simulink model "GFo_29bus"  (R2015b)
settings: Solver=ode1  StartTime=0.0  StopTime=4.5  FixedStep=Time_Step  RelTol=1e-3
PreLoadFcn:
  | Init_29bus;
InitFcn:
  | Init_29bus;
undefined symbols (not defined in the file): C_line, D1, D11, Delta, DX_DR, fb, fn, I_thresh_pu, Kp_Rvi_pu, Time_Step, VSC01_Cf, VSC01_Cf_pu, VSC01_Delta_P_Time_Step, VSC01_Delta_P_Value, VSC01_id0, VSC01_Lf, VSC01_Lf_pu, VSC01_Lt_pu, VSC01_mp1, VSC01_mp2, VSC01_mp3, VSC01_Pn, VSC01_R, VSC01_Rf, VSC01_Rf_pu, VSC01_Rt_pu, VSC01_Rv, VSC01_Sn, VSC01_T1, VSC01_T2, VSC01_Tr_PLL, VSC01_Udc_n, VSC01_Udcb, VSC01_Un1, VSC01_Un2, VSC01_W_LF, VSC01_wc1, VSC01_wc2, VSC01_wc3
libraries: powerlib x183, sps_avr x6, simulink x4, powerlib_meascontrol x2
(part 5 of 6)

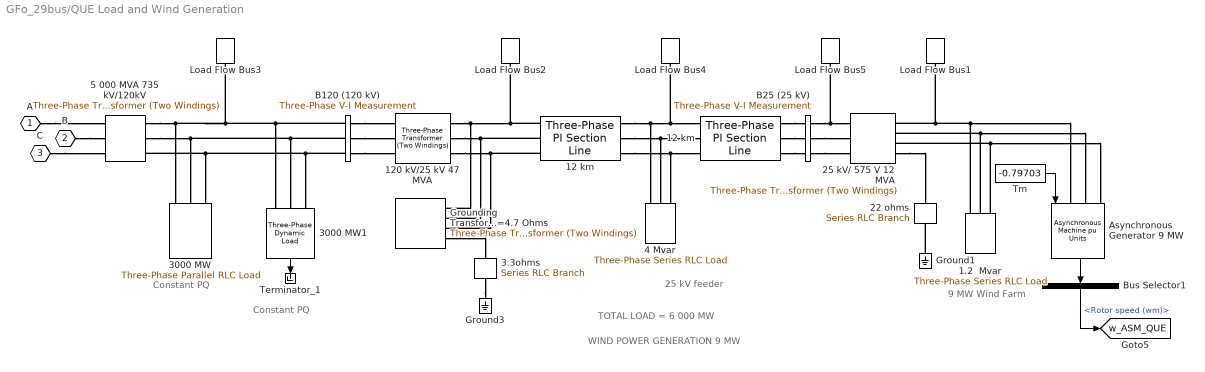
== system GFo_29bus/QUE Load and Wind Generation ==
  note: 9 MW Wind Farm
  note: 25 kV feeder
  note: Constant PQ
  note: Constant PQ
  note: WIND POWER GENERATION 9 MW
  note: TOTAL LOAD = 6 000 MW
  1.2  Mvar : powerlib/Elements/Three-Phase Series RLC Load  LConnTagsString=A|B|C  Configuration=Delta  NominalVoltage=575  Vabc=[1e3 1e3 1e3]  Vabcp=[1e3 1e3 1e3]  NominalFrequency=60  UnbalancedPower=off  ActivePower=1.2e6/50  InductivePower=0  CapacitivePower=1.2e6  Pabc=[10e3 9e3 11e3]  QLabc=[100 90 110]  QCabc=[100 90 110]  Pabcp=[10e3 9e3 11e3]  QLabcp=[100 90 110]  QCabcp=[100 90 110]  Measurements=None  LoadType=constant Z
  12 km : powerlib/Elements/Three-Phase PI Section Line  LConnTagsString=a|b|c  RConnTagsString=A|B|C  Frequency=60  Resistances=[0.1153 0.413]  Inductances=[1.05e-3 3.32e-3]  Capacitances=[11.33e-009 5.01e-009]  Length=12
  "12 km " : powerlib/Elements/Three-Phase PI Section Line  LConnTagsString=a|b|c  RConnTagsString=A|B|C  Frequency=60  Resistances=[0.1153 0.413]  Inductances=[1.05e-3 3.32e-3]  Capacitances=[11.33e-009 5.01e-009]  Length=12
  120 kV/25 kV 47 MVA : powerlib/Elements/Three-Phase Transformer (Two Windings)  Winding1Connection=Yg  Winding2Connection=Delta (D1)  CoreType=Three single-phase transformers  SetSaturation=off  Hysteresis=off  DataFile='basic_model'  SetInitialFlux=off  Measurements=None  UNITS=pu  NominalPower=[47e6 60 ]  Winding1="[ 120e3  0.08/30   0.08 ]"  Winding2="[ 25e3  0.08/30  0.08]"  Rm=500  Lm=500  L0=0.5  Saturation="[ 0,0  ;  0.005,1.2  ;  1.0,1.4 ]"  InitialFluxes=[ 0.8 , -0.8 , 0.7 ]  MoreParameters=off  BreakLoop=off  DataType=off  TransfoNumber=0
  "22 ohms " : powerlib/Elements/Series RLC Branch  LConnTagsString=__new0  RConnTagsString=__new0  BranchType=R  Resistance=22  Inductance=1.0  SetiL0=off  InitialCurrent=0  Capacitance=1.0  Setx0=off  InitialVoltage=0  Measurements=None
  25 kV/ 575 V 12 MVA : powerlib/Elements/Three-Phase Transformer (Two Windings)  Winding1Connection=Yg  Winding2Connection=Yn  CoreType=Three single-phase transformers  SetSaturation=off  Hysteresis=off  DataFile='hysteresis'  SetInitialFlux=off  Measurements=None  UNITS=pu  NominalPower="[12e6  60]"  Winding1=[25e3 , 0.025/30 , 0.025]  Winding2=[ 575, 0.025/30 , 0.025]  Rm=500  Lm=inf  L0=0.5  Saturation=[ 0,0 ; 0.0024,1.2 ; 1.0,1.52 ]  InitialFluxes=[ 0.8 , -0.8 , 0.7 ]  MoreParameters=off  BreakLoop=off  DataType=off  TransfoNumber=0
  "3.3ohms " : powerlib/Elements/Series RLC Branch  LConnTagsString=__new0  RConnTagsString=__new0  BranchType=R  Resistance=3.3  Inductance=1.0  SetiL0=off  InitialCurrent=0  Capacitance=1.0  Setx0=off  InitialVoltage=0  Measurements=None
  3000 MW : powerlib/Elements/Three-Phase Parallel RLC Load  LConnTagsString=A|B|C  Configuration=Y (grounded)  NominalVoltage=(120000)*1.00073  Vabc=[1e3 1e3 1e3]  Vabcp=[1e3 1e3 1e3]  NominalFrequency=60  UnbalancedPower=off  ActivePower=3000000000  InductivePower=0  CapacitivePower=0  Pabc=[10e3 9e3 11e3]  QLabc=[100 90 110]  QCabc=[100 90 110]  Pabcp=[10e3 9e3 11e3]  QLabcp=[100 90 110]  QCabcp=[100 90 110]  Measurements=None  LoadType=constant PQ
  3000 MW1 : powerlib/Elements/Three-Phase Dynamic Load  NominalVoltage=[ 120e3 60 ]  ActiveReactivePowers=[3e+09 -3.55271e-07]  PositiveSequence=[1.00073 -50.5771]  ExternalControl=off  NpNq=[1.3 2]  TimeConstants="[0  0  0  0]"  MinimumVoltage=0.7  Tfilter=1e-4  LoadFlowParameters=[4,0,0,0,0]
  4 Mvar : powerlib/Elements/Three-Phase Series RLC Load  LConnTagsString=A|B|C  Configuration=Delta  NominalVoltage=25e3  Vabc=[1e3 1e3 1e3]  Vabcp=[1e3 1e3 1e3]  NominalFrequency=60  UnbalancedPower=off  ActivePower=0  InductivePower=0  CapacitivePower=4e6  Pabc=[10e3 9e3 11e3]  QLabc=[100 90 110]  QCabc=[100 90 110]  Pabcp=[10e3 9e3 11e3]  QLabcp=[100 90 110]  QCabcp=[100 90 110]  Measurements=None  LoadType=constant Z
  5 000 MVA 735 kV/120kV : powerlib/Elements/Three-Phase Transformer (Two Windings)  Winding1Connection=Yg  Winding2Connection=Delta (D1)  CoreType=Three single-phase transformers  SetSaturation=off  Hysteresis=off  DataFile='basic_model'  SetInitialFlux=off  Measurements=None  UNITS=pu  NominalPower=[ 5000e6 60 ]  Winding1="[ 735e3 0.002  0.12]"  Winding2=[120e3 0.002 0]  Rm=500  Lm=500  L0=0.5  Saturation="[ 0,0  ;  0.005,1.2  ;  1.0,1.4 ]"  InitialFluxes=[ 0.8 , -0.8 , 0.7 ]  MoreParameters=off  BreakLoop=off  DataType=off  TransfoNumber=0
  Asynchronous Generator 9 MW : powerlib/Machines/Asynchronous Machine pu Units  RotorType=Squirrel-cage  PresetModel=No  MechanicalLoad=Torque Tm  ShowDetailedParameters=on  ReferenceFrame=Rotor  Units=pu  MeasurementBus=off  NominalParameters=[6*1.5e6/0.9 575 60]  Stator=[ 0.004843 0.1248]  Rotor=[ 0.004377 0.1791]  Cage1=[0.01909 0.0397]  Cage2=[0.01909 0.0397]  Lm=6.77  Mechanical="[5.04  0  3]"  PolePairs=3  InitialConditions=[-0.00372401 0 0.857274 0.857274 0.857274 133.477 13.4769 253.477]  SimulateSaturation=off  Saturation=[ 0 0 ; 0 0 ]  LoadFlowParameters=0  TsPowergui=0  TsBlock=-1  IterativeModel=Trapezoidal non iterative  IterativeDiscreteModel=Trapezoidal non iterative  Pmec=-8000000
  B120 (120 kV) : powerlib/Measurements/Three-Phase V-I Measurement  VoltageMeasurement=no  SetLabelV=on  LabelV=Vabc_B120  Vpu=on  VpuLL=off  CurrentMeasurement=no  SetLabelI=on  LabelI=Iabc_B120  Ipu=off  Pbase=100e6  Vbase=120e3  OutputType=Complex  PhasorSimulation=off  PSBequivalent=0
  B25 (25 kV) : powerlib/Measurements/Three-Phase V-I Measurement  VoltageMeasurement=no  SetLabelV=on  LabelV=Vabc_B25  Vpu=on  VpuLL=off  CurrentMeasurement=no  SetLabelI=on  LabelI=Iabc_B25  Ipu=on  Pbase=10e6  Vbase=25e3  OutputType=Complex  PhasorSimulation=off  PSBequivalent=0
  Bus Selector1 : BusSelector  OutputSignals=Mechanical.Rotor speed (wm)
  Ground1 : powerlib/Elements/Ground  LConnTagsString=a
  Ground3 : powerlib/Elements/Ground  LConnTagsString=a
  Grounding Transformer X0=4.7 Ohms : powerlib/Elements/Three-Phase Transformer (Two Windings)  Winding1Connection=Yn  Winding2Connection=Delta (D11)  CoreType=Three single-phase transformers  SetSaturation=off  Hysteresis=off  DataFile='basic_model'  SetInitialFlux=off  Measurements=None  UNITS=pu  NominalPower=[100e6 60]  Winding1="[ 25e3  4.7/(25e3^2/100e6)/30    4.7/(25e3^2/100e6)]"  Winding2="[ 25e3  1e-6  0]"  Rm=500  Lm=500  L0=0.5  Saturation="[ 0,0  ;  0.005,1.2  ;  1.0,1.4 ]"  InitialFluxes=[ 0.8 , -0.8 , 0.7 ]  MoreParameters=off  BreakLoop=off  DataType=off  TransfoNumber=0
  Load Flow Bus1 : powerlib/Measurements/Load Flow Bus  LConnTagsString=a  Phases=single  Connectors=on one side  ID=QUE_575  Vbase=575  Vref=1  Vangle=0  VLF=1.014  VLFb=1  VLFc=1  angleLF=-70.61  angleLFb=0  angleLFc=0
      settings: AttributesFormatString=%<ID>\n%<Vbase>V\n%<VLF>pu\n%<angleLF>deg.
  Load Flow Bus2 : powerlib/Measurements/Load Flow Bus  LConnTagsString=a  Phases=single  Connectors=on one side  ID=QUE_25_1  Vbase=25e3  Vref=1  Vangle=0  VLF=1.003  VLFb=1  VLFc=1  angleLF=-79.15  angleLFb=0  angleLFc=0
      settings: AttributesFormatString=%<ID>\n%<Vbase>V\n%<VLF>pu\n%<angleLF>deg.
  Load Flow Bus3 : powerlib/Measurements/Load Flow Bus  LConnTagsString=a  Phases=single  Connectors=on one side  ID=QUE1  Vbase=120e3  Vref=1  Vangle=0  VLF=1.001  VLFb=1  VLFc=1  angleLF=-50.58  angleLFb=0  angleLFc=0
      settings: AttributesFormatString=%<ID>\n%<Vbase>V\n%<VLF>pu\n%<angleLF>deg.
  Load Flow Bus4 : powerlib/Measurements/Load Flow Bus  LConnTagsString=a  Phases=single  Connectors=on one side  ID=QUE_25_2  Vbase=25e3  Vref=1  Vangle=0  VLF=1.027  VLFb=1  VLFc=1  angleLF=-76.03  angleLFb=0  angleLFc=0
      settings: AttributesFormatString=%<ID>\n%<Vbase>V\n%<VLF>pu\n%<angleLF>deg.
  Load Flow Bus5 : powerlib/Measurements/Load Flow Bus  LConnTagsString=a  Phases=single  Connectors=on one side  ID=QUE_25_3  Vbase=25e3  Vref=1  Vangle=0  VLF=1.023  VLFb=1  VLFc=1  angleLF=-72.45  angleLFb=0  angleLFc=0
      settings: AttributesFormatString=%<ID>\n%<Vbase>V\n%<VLF>pu\n%<angleLF>deg.
  Terminator_1 : Terminator
  Tm : Constant  Value=-0.79703
  A : PMIOPort  Port=1  Side=Left
  B : PMIOPort  Port=2  Side=Left
  C : PMIOPort  Port=3  Side=Left
  tag scope: w_ASM_QUE=global
  wires:
  Tm/1 -> Asynchronous Generator 9 MW/1
  Asynchronous Generator 9 MW/1 -> Bus Selector1/1
  Bus Selector1/1 -> [w_ASM_QUE]  "<Rotor speed (wm)>"
  3000 MW1/1 -> Terminator_1/1
  connections:
  B120 (120 kV)/RConn3 -- 120 kV/25 kV 47 MVA/LConn3
  B120 (120 kV)/RConn2 -- 120 kV/25 kV 47 MVA/LConn2
  B120 (120 kV)/RConn1 -- 120 kV/25 kV 47 MVA/LConn1
  A/RConn1 -- 5 000 MVA 735 kV/120kV/LConn1
  B/RConn1 -- 5 000 MVA 735 kV/120kV/LConn2
  C/RConn1 -- 5 000 MVA 735 kV/120kV/LConn3
  Load Flow Bus3/LConn1 -- B120 (120 kV)/LConn1 -- 3000 MW1/LConn1 -- 5 000 MVA 735 kV/120kV/RConn1 -- 3000 MW/LConn1
  B120 (120 kV)/LConn2 -- 5 000 MVA 735 kV/120kV/RConn2 -- 3000 MW/LConn2 -- 3000 MW1/LConn2
  B120 (120 kV)/LConn3 -- 5 000 MVA 735 kV/120kV/RConn3 -- 3000 MW/LConn3 -- 3000 MW1/LConn3
  12 km/LConn2 -- 120 kV/25 kV 47 MVA/RConn2 -- Grounding Transformer X0=4.7 Ohms/LConn2
  12 km/LConn3 -- 120 kV/25 kV 47 MVA/RConn3 -- Grounding Transformer X0=4.7 Ohms/LConn3
  Load Flow Bus2/LConn1 -- 12 km/LConn1 -- Grounding Transformer X0=4.7 Ohms/LConn1 -- 120 kV/25 kV 47 MVA/RConn1
  "3.3ohms "/RConn1 -- Ground3/LConn1
  Grounding Transformer X0=4.7 Ohms/LConn4 -- "3.3ohms "/LConn1
  25 kV/ 575 V 12 MVA/RConn4 -- "22 ohms "/LConn1
  Ground1/LConn1 -- "22 ohms "/RConn1
  Load Flow Bus1/LConn1 -- 1.2  Mvar/LConn1 -- Asynchronous Generator 9 MW/LConn1 -- 25 kV/ 575 V 12 MVA/RConn1
  1.2  Mvar/LConn2 -- 25 kV/ 575 V 12 MVA/RConn2 -- Asynchronous Generator 9 MW/LConn2
  1.2  Mvar/LConn3 -- 25 kV/ 575 V 12 MVA/RConn3 -- Asynchronous Generator 9 MW/LConn3
  B25 (25 kV)/RConn1 -- 25 kV/ 575 V 12 MVA/LConn1 -- Load Flow Bus5/LConn1
  B25 (25 kV)/RConn2 -- 25 kV/ 575 V 12 MVA/LConn2
  B25 (25 kV)/RConn3 -- 25 kV/ 575 V 12 MVA/LConn3
  "12 km "/RConn1 -- B25 (25 kV)/LConn1
  "12 km "/RConn2 -- B25 (25 kV)/LConn2
  "12 km "/RConn3 -- B25 (25 kV)/LConn3
  12 km/RConn1 -- "12 km "/LConn1 -- Load Flow Bus4/LConn1 -- 4 Mvar/LConn1
  12 km/RConn2 -- "12 km "/LConn2 -- 4 Mvar/LConn2
  12 km/RConn3 -- "12 km "/LConn3 -- 4 Mvar/LConn3

== system GFo_29bus/Subsystem ==
  Ground_1 : Ground
  Mux : Mux  Inputs=6
  Mux1 : Mux  Inputs=6
  "SM speeds yel=LG2 mag=LG3 cyan=LG4 red=MTL green=CHU blue=MAN " : Scope
  SM terminal voltages yel=LG2 mag=LG3 cyan=LG4 red=MTL green=CHU blue=MAN : Scope
  Scope : Scope
  Scope1 : Scope
  wires:
  [Vabc_MTL7] -> Scope/1
  [w_ASM_QUE] -> Scope1/1
  Mux/1 -> "SM speeds yel=LG2 mag=LG3 cyan=LG4 red=MTL green=CHU blue=MAN "/1  "w (pu)"
  [w1] -> Mux/1
  [w2] -> Mux/2
  [w7] -> Mux/6
  [w6] -> Mux/5
  [w3] -> Mux/3
  Mux1/1 -> SM terminal voltages yel=LG2 mag=LG3 cyan=LG4 red=MTL green=CHU blue=MAN/1  "Vm (pu)"
  [Vm1] -> Mux1/1
  [Vm2] -> Mux1/2
  [Vm7] -> Mux1/6
  [Vm6] -> Mux1/5
  [Vm4] -> Mux1/4
  [Vm3] -> Mux1/3
  Ground_1/1 -> Mux/4

== system GFo_29bus/Subsystem1 ==
  In1 : Inport
  Constant : Constant
  Sum : Sum  Inputs=|++  SaturateOnIntegerOverflow=on
  tag scope: PSS_select=global
  wires:
  In1/1 -> Sum/1
  Sum/1 -> [PSS_select]
  Constant/1 -> Sum/2

== system GFo_29bus/Subsystem2 ==

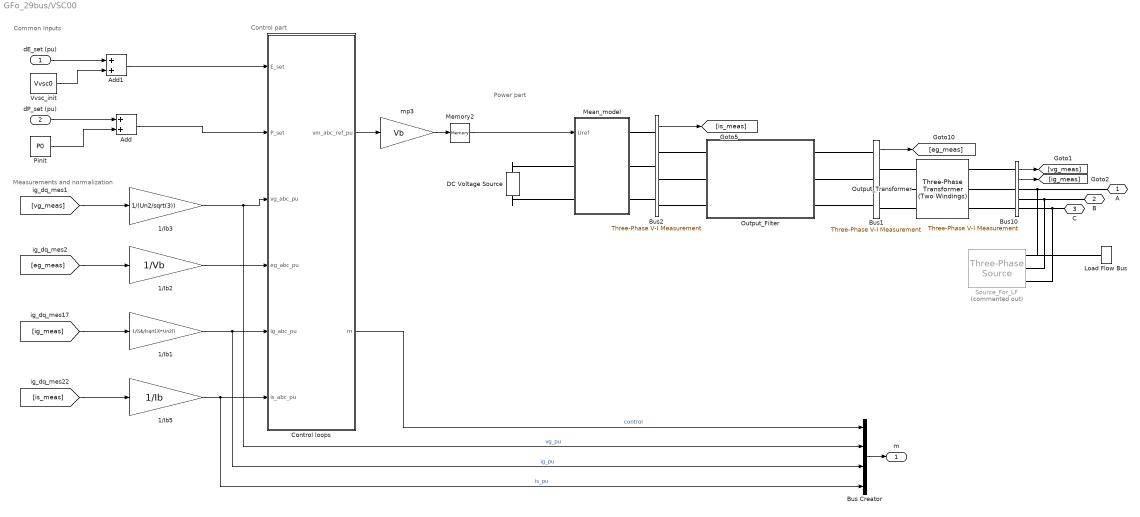
== system GFo_29bus/VSC00 ==
  note: Control part
  note: Measurements and normalization
  note: Power part
  note: Common Inputs
  dE_set (pu) : Inport
  dP_set (pu) : Inport  Port=2
  1/Ib1 : Gain  Gain=1/(Sb/(sqrt(3)*Un2))
  1/Ib2 : Gain  Gain=1/Vb
  1/Ib3 : Gain  Gain=1/(Un2/sqrt(3))
  1/Ib5 : Gain  Gain=1/Ib
  Add : Sum
  Add1 : Sum
  Bus Creator : BusCreator  Inputs=4
  Bus1 : powerlib/Measurements/Three-Phase V-I Measurement  VoltageMeasurement=phase-to-ground  SetLabelV=off  LabelV=Vabc  Vpu=off  VpuLL=off  CurrentMeasurement=no  SetLabelI=off  LabelI=Iabc  Ipu=off  Pbase=100e6  Vbase=500e3  OutputType=Complex  PhasorSimulation=off  PSBequivalent=0
  Bus10 : powerlib/Measurements/Three-Phase V-I Measurement  VoltageMeasurement=phase-to-ground  SetLabelV=off  LabelV=Vabc  Vpu=off  VpuLL=off  CurrentMeasurement=yes  SetLabelI=off  LabelI=Iabc  Ipu=off  Pbase=100e6  Vbase=500e3  OutputType=Complex  PhasorSimulation=off  PSBequivalent=0
  Bus2 : powerlib/Measurements/Three-Phase V-I Measurement  VoltageMeasurement=no  SetLabelV=off  LabelV=Vabc  Vpu=off  VpuLL=off  CurrentMeasurement=yes  SetLabelI=off  LabelI=Iabc  Ipu=off  Pbase=100e6  Vbase=500e3  OutputType=Complex  PhasorSimulation=off  PSBequivalent=0
  Control loops : Subsystem
  DC Voltage Source : powerlib/Electrical Sources/DC Voltage Source  Amplitude=VSC01_Udc_n  Measurements=Voltage
  Load Flow Bus : powerlib/Measurements/Load Flow Bus  LConnTagsString=a  Phases=single  Connectors=on one side  ID=VSC00  Vbase=Un2  Vref=V0  Vangle=Theta0  VLF=1  VLFb=1  VLFc=1  angleLF=-20.98  angleLFb=0  angleLFc=0
  Mean_model : Subsystem
  Memory2 : Memory  X0=[Va0 Vb0 Vc0]
  Output_Filter : Subsystem  mask{Lf=VSC01_Lf, Rf=VSC01_Rf, Cf=VSC01_Cf}
      mask prompts: Lf "Filter inductance [H]"; Rf "Filter resistance [R]"; Cf "Filter capacitance [F]"
  Output_Transformer : powerlib/Elements/Three-Phase Transformer (Two Windings)  Winding1Connection=Yg  Winding2Connection=Yg  CoreType=Three single-phase transformers  SetSaturation=off  Hysteresis=off  DataFile='hysteresis'  SetInitialFlux=off  Measurements=None  UNITS=pu  NominalPower=[Sn , fn ]  Winding1=[Un1 , Rt_pu/2 , Lt_pu/2]  Winding2=[Un2 , Rt_pu/2 , Lt_pu/2]  Rm=Rm_pu  Lm=Lm_pu  L0=0.5  Saturation=[ 0,0 ; 0.0024,1.2 ; 1.0,1.52 ]  InitialFluxes=[-1.0109960716468 0.506091473811006 0.504904597835851]  MoreParameters=off  BreakLoop=off  DataType=off  TransfoNumber=1
  Pinit : Constant  Value=P0
  Source_For_LF : powerlib/Electrical Sources/Three-Phase Source  Commented=on  InternalConnection=Yg  VoltagePhases=off  Voltage=(735000)*1  PhaseAngle=-20.9762  Voltage_phases=[25e3 25e3 25e3]/sqrt(3)  PhaseAngles_phases=[0 -120 +120]  Frequency=fb  NonIdealSource=off  SpecifyImpedance=off  Resistance=0  Inductance=0  ShortCircuitLevel=100e6  BaseVoltage=Un  XRratio=7  BusType=PV  Pref=P0*Sb  Qref=Q0*Sb  Prefabc=[10e3, 10e3, 10e3]  Qrefabc=[0, 0, 0]  Qmin=-inf  Qmax=inf
  Vvsc_init : Constant  Value=Vvsc0
  mp3 : Gain  Gain=Vb
  A : PMIOPort  Port=1  Side=Right
  B : PMIOPort  Port=2  Side=Right
  C : PMIOPort  Port=3  Side=Right
  m : Outport
  wires:
  Add/1 -> Control loops/2(P_set)
  dE_set (pu)/1 -> Add1/1
  Bus1/1 -> [eg_meas]
  Add1/1 -> Control loops/1(E_set)
  Vvsc_init/1 -> Add1/2
  Pinit/1 -> Add/2
  dP_set (pu)/1 -> Add/1
  Bus10/1 -> [vg_meas]
  Bus2/1 -> [is_meas]
  Memory2/1 -> Mean_model/1(Uref)
  Bus10/2 -> [ig_meas]
  [is_meas] -> 1/Ib5/1
  1/Ib1/1 -> Control loops/5(ig_abc_pu), Bus Creator/3  "ig_pu"
  [ig_meas] -> 1/Ib1/1
  [vg_meas] -> 1/Ib3/1
  1/Ib3/1 -> Bus Creator/2, Control loops/3(vg_abc_pu)  "vg_pu"
  Control loops/2(m) -> Bus Creator/1  "control"
  Bus Creator/1 -> m/1
  [eg_meas] -> 1/Ib2/1
  1/Ib2/1 -> Control loops/4(eg_abc_pu)
  1/Ib5/1 -> Control loops/6(is_abc_pu), Bus Creator/4  "is_pu"
  Control loops/1(vm_abc_ref_pu) -> mp3/1
  mp3/1 -> Memory2/1
  connections:
  DC Voltage Source/RConn1 -- Mean_model/LConn1
  DC Voltage Source/LConn1 -- Mean_model/LConn2
  Bus1/LConn1 -- Output_Filter/RConn1
  Bus1/LConn2 -- Output_Filter/RConn2
  Bus1/LConn3 -- Output_Filter/RConn3
  Output_Transformer/LConn1 -- Bus1/RConn1
  Bus1/RConn2 -- Output_Transformer/LConn2
  Bus1/RConn3 -- Output_Transformer/LConn3
  Bus10/LConn1 -- Output_Transformer/RConn1
  Bus10/LConn2 -- Output_Transformer/RConn2
  Bus10/LConn3 -- Output_Transformer/RConn3
  C/RConn1 -- Source_For_LF/RConn3 -- Bus10/RConn3
  B/RConn1 -- Source_For_LF/RConn2 -- Bus10/RConn2
  A/RConn1 -- Load Flow Bus/LConn1 -- Source_For_LF/RConn1 -- Bus10/RConn1
  Bus2/LConn1 -- Mean_model/RConn1
  Bus2/LConn2 -- Mean_model/RConn2
  Bus2/LConn3 -- Mean_model/RConn3
  Bus2/RConn1 -- Output_Filter/LConn1
  Bus2/RConn2 -- Output_Filter/LConn2
  Bus2/RConn3 -- Output_Filter/LConn3

== system GFo_29bus/North-West Network/Cs  CHMN  ==
  note: B
  Ca : powerlib/Elements/Series RLC Branch  LConnTagsString=__new0  RConnTagsString=__new0  BranchType=C  Resistance=1.0  Inductance=1.0  SetiL0=off  InitialCurrent=0  Capacitance=Cs  Setx0=off  InitialVoltage=0  Measurements=None
  Cb : powerlib/Elements/Series RLC Branch  LConnTagsString=__new0  RConnTagsString=__new0  BranchType=C  Resistance=1.0  Inductance=1.0  SetiL0=off  InitialCurrent=0  Capacitance=Cs  Setx0=off  InitialVoltage=0  Measurements=None
  Cc : powerlib/Elements/Series RLC Branch  LConnTagsString=__new0  RConnTagsString=__new0  BranchType=C  Resistance=1.0  Inductance=1.0  SetiL0=off  InitialCurrent=0  Capacitance=Cs  Setx0=off  InitialVoltage=0  Measurements=None
  A : PMIOPort  Port=1  Side=Left
  B : PMIOPort  Port=2  Side=Left
  C : PMIOPort  Port=3  Side=Left
  "A " : PMIOPort  Port=4  Side=Right
  "B " : PMIOPort  Port=5  Side=Right
  "C " : PMIOPort  Port=6  Side=Right
  connections:
  Cc/RConn1 -- "C "/RConn1
  C/RConn1 -- Cc/LConn1
  Cb/RConn1 -- "B "/RConn1
  B/RConn1 -- Cb/LConn1
  Ca/RConn1 -- "A "/RConn1
  A/RConn1 -- Ca/LConn1

== system GFo_29bus/North-West Network/Cs ABI+CHB  ==
  note: B
  Ca : powerlib/Elements/Series RLC Branch  LConnTagsString=__new0  RConnTagsString=__new0  BranchType=C  Resistance=1.0  Inductance=1.0  SetiL0=off  InitialCurrent=0  Capacitance=Cs  Setx0=off  InitialVoltage=0  Measurements=None
  Cb : powerlib/Elements/Series RLC Branch  LConnTagsString=__new0  RConnTagsString=__new0  BranchType=C  Resistance=1.0  Inductance=1.0  SetiL0=off  InitialCurrent=0  Capacitance=Cs  Setx0=off  InitialVoltage=0  Measurements=None
  Cc : powerlib/Elements/Series RLC Branch  LConnTagsString=__new0  RConnTagsString=__new0  BranchType=C  Resistance=1.0  Inductance=1.0  SetiL0=off  InitialCurrent=0  Capacitance=Cs  Setx0=off  InitialVoltage=0  Measurements=None
  A : PMIOPort  Port=1  Side=Left
  B : PMIOPort  Port=2  Side=Left
  C : PMIOPort  Port=3  Side=Left
  "A " : PMIOPort  Port=4  Side=Right
  "B " : PMIOPort  Port=5  Side=Right
  "C " : PMIOPort  Port=6  Side=Right
  connections:
  Cc/RConn1 -- "C "/RConn1
  C/RConn1 -- Cc/LConn1
  Cb/RConn1 -- "B "/RConn1
  B/RConn1 -- Cb/LConn1
  Ca/RConn1 -- "A "/RConn1
  A/RConn1 -- Ca/LConn1

== system GFo_29bus/North-West Network/Cs ALB ==
  note: B
  Ca : powerlib/Elements/Series RLC Branch  LConnTagsString=__new0  RConnTagsString=__new0  BranchType=C  Resistance=1.0  Inductance=1.0  SetiL0=off  InitialCurrent=0  Capacitance=Cs  Setx0=off  InitialVoltage=0  Measurements=None
  Cb : powerlib/Elements/Series RLC Branch  LConnTagsString=__new0  RConnTagsString=__new0  BranchType=C  Resistance=1.0  Inductance=1.0  SetiL0=off  InitialCurrent=0  Capacitance=Cs  Setx0=off  InitialVoltage=0  Measurements=None
  Cc : powerlib/Elements/Series RLC Branch  LConnTagsString=__new0  RConnTagsString=__new0  BranchType=C  Resistance=1.0  Inductance=1.0  SetiL0=off  InitialCurrent=0  Capacitance=Cs  Setx0=off  InitialVoltage=0  Measurements=None
  A : PMIOPort  Port=1  Side=Left
  B : PMIOPort  Port=2  Side=Left
  C : PMIOPort  Port=3  Side=Left
  "A " : PMIOPort  Port=4  Side=Right
  "B " : PMIOPort  Port=5  Side=Right
  "C " : PMIOPort  Port=6  Side=Right
  connections:
  A/RConn1 -- Ca/LConn1
  Ca/RConn1 -- "A "/RConn1
  B/RConn1 -- Cb/LConn1
  Cb/RConn1 -- "B "/RConn1
  C/RConn1 -- Cc/LConn1
  Cc/RConn1 -- "C "/RConn1

== system GFo_29bus/North-West Network/Cs LVDN  ==
  note: B
  Ca : powerlib/Elements/Series RLC Branch  LConnTagsString=__new0  RConnTagsString=__new0  BranchType=C  Resistance=1.0  Inductance=1.0  SetiL0=off  InitialCurrent=0  Capacitance=Cs  Setx0=off  InitialVoltage=0  Measurements=None
  Cb : powerlib/Elements/Series RLC Branch  LConnTagsString=__new0  RConnTagsString=__new0  BranchType=C  Resistance=1.0  Inductance=1.0  SetiL0=off  InitialCurrent=0  Capacitance=Cs  Setx0=off  InitialVoltage=0  Measurements=None
  Cc : powerlib/Elements/Series RLC Branch  LConnTagsString=__new0  RConnTagsString=__new0  BranchType=C  Resistance=1.0  Inductance=1.0  SetiL0=off  InitialCurrent=0  Capacitance=Cs  Setx0=off  InitialVoltage=0  Measurements=None
  A : PMIOPort  Port=1  Side=Left
  B : PMIOPort  Port=2  Side=Left
  C : PMIOPort  Port=3  Side=Left
  "A " : PMIOPort  Port=4  Side=Right
  "B " : PMIOPort  Port=5  Side=Right
  "C " : PMIOPort  Port=6  Side=Right
  connections:
  A/RConn1 -- Ca/LConn1
  Ca/RConn1 -- "A "/RConn1
  B/RConn1 -- Cb/LConn1
  Cb/RConn1 -- "B "/RConn1
  C/RConn1 -- Cc/LConn1
  Cc/RConn1 -- "C "/RConn1

== system GFo_29bus/North-West Network/Cs LVDS  ==
  note: B
  Ca : powerlib/Elements/Series RLC Branch  LConnTagsString=__new0  RConnTagsString=__new0  BranchType=C  Resistance=1.0  Inductance=1.0  SetiL0=off  InitialCurrent=0  Capacitance=Cs  Setx0=off  InitialVoltage=0  Measurements=None
  Cb : powerlib/Elements/Series RLC Branch  LConnTagsString=__new0  RConnTagsString=__new0  BranchType=C  Resistance=1.0  Inductance=1.0  SetiL0=off  InitialCurrent=0  Capacitance=Cs  Setx0=off  InitialVoltage=0  Measurements=None
  Cc : powerlib/Elements/Series RLC Branch  LConnTagsString=__new0  RConnTagsString=__new0  BranchType=C  Resistance=1.0  Inductance=1.0  SetiL0=off  InitialCurrent=0  Capacitance=Cs  Setx0=off  InitialVoltage=0  Measurements=None
  A : PMIOPort  Port=1  Side=Left
  B : PMIOPort  Port=2  Side=Left
  C : PMIOPort  Port=3  Side=Left
  "A " : PMIOPort  Port=4  Side=Right
  "B " : PMIOPort  Port=5  Side=Right
  "C " : PMIOPort  Port=6  Side=Right
  connections:
  Cc/RConn1 -- "C "/RConn1
  C/RConn1 -- Cc/LConn1
  Cb/RConn1 -- "B "/RConn1
  B/RConn1 -- Cb/LConn1
  Ca/RConn1 -- "A "/RConn1
  A/RConn1 -- Ca/LConn1

== system GFo_29bus/North-West Network/Cs NEM  ==
  note: B
  Ca : powerlib/Elements/Series RLC Branch  LConnTagsString=__new0  RConnTagsString=__new0  BranchType=C  Resistance=1.0  Inductance=1.0  SetiL0=off  InitialCurrent=0  Capacitance=Cs  Setx0=off  InitialVoltage=0  Measurements=None
  Cb : powerlib/Elements/Series RLC Branch  LConnTagsString=__new0  RConnTagsString=__new0  BranchType=C  Resistance=1.0  Inductance=1.0  SetiL0=off  InitialCurrent=0  Capacitance=Cs  Setx0=off  InitialVoltage=0  Measurements=None
  Cc : powerlib/Elements/Series RLC Branch  LConnTagsString=__new0  RConnTagsString=__new0  BranchType=C  Resistance=1.0  Inductance=1.0  SetiL0=off  InitialCurrent=0  Capacitance=Cs  Setx0=off  InitialVoltage=0  Measurements=None
  A : PMIOPort  Port=1  Side=Left
  B : PMIOPort  Port=2  Side=Left
  C : PMIOPort  Port=3  Side=Left
  "A " : PMIOPort  Port=4  Side=Right
  "B " : PMIOPort  Port=5  Side=Right
  "C " : PMIOPort  Port=6  Side=Right
  connections:
  A/RConn1 -- Ca/LConn1
  Ca/RConn1 -- "A "/RConn1
  B/RConn1 -- Cb/LConn1
  Cb/RConn1 -- "B "/RConn1
  C/RConn1 -- Cc/LConn1
  Cc/RConn1 -- "C "/RConn1

== system GFo_29bus/North-West Network/Regulators1 ==
  m : Inport
  Bus Selector1 : BusSelector  OutputSignals="dq0 components.Stator voltage  vq (pu),dq0 components.Stator voltage  vd (pu),Mechanical.Rotor speed  wm  (pu),Output active power   Peo (pu)"
  Math Function1 : Math  Operator=hypot  SaturateOnIntegerOverflow=on
  Pref1 : Constant
  Turbine  & Excitation Regulators Mac2 : Subsystem
  Vref : Constant  Value=0.90977
  Pm : Outport
  Vf : Outport  Port=2
  tag scope: Vm1=global, w1=global
  wires:
  Pref1/1 -> Turbine  & Excitation Regulators Mac2/2(Vref)
  Turbine  & Excitation Regulators Mac2/1(Pm) -> Pm/1
  Vref/1 -> Turbine  & Excitation Regulators Mac2/1(Pref)
  Turbine  & Excitation Regulators Mac2/2(Vf) -> Vf/1
  Bus Selector1/1 -> Math Function1/1  "<Stator voltage  vq (pu)>"
  Bus Selector1/2 -> Math Function1/2  "<Stator voltage  vd (pu)>"
  Math Function1/1 -> Turbine  & Excitation Regulators Mac2/3(Vm), [Vm1]
  Bus Selector1/3 -> Turbine  & Excitation Regulators Mac2/4(w), [w1]  "<Rotor speed  wm  (pu)>"
  Bus Selector1/4 -> Turbine  & Excitation Regulators Mac2/5(Pe)  "<Output active power   Peo (pu)>"
  m/1 -> Bus Selector1/1

== system GFo_29bus/North-West Network/Regulators2 ==
  m : Inport
  Bus Selector1 : BusSelector  OutputSignals="dq0 components.Stator voltage  vq (pu),dq0 components.Stator voltage  vd (pu),Mechanical.Rotor speed  wm  (pu),Output active power   Peo (pu)"
  Math Function1 : Math  Operator=hypot  SaturateOnIntegerOverflow=on
  Pref1 : Constant
  Turbine  & Excitation Regulators Mac2 : Subsystem
  Vref : Constant  Value=0.81818
  Pm : Outport
  Vf : Outport  Port=2
  tag scope: Vm2=global, w2=global
  wires:
  m/1 -> Bus Selector1/1
  Bus Selector1/4 -> Turbine  & Excitation Regulators Mac2/5(Pe)  "<Output active power   Peo (pu)>"
  Bus Selector1/3 -> [w2], Turbine  & Excitation Regulators Mac2/4(w)  "<Rotor speed  wm  (pu)>"
  Math Function1/1 -> [Vm2], Turbine  & Excitation Regulators Mac2/3(Vm)
  Bus Selector1/2 -> Math Function1/2  "<Stator voltage  vd (pu)>"
  Bus Selector1/1 -> Math Function1/1  "<Stator voltage  vq (pu)>"
  Turbine  & Excitation Regulators Mac2/2(Vf) -> Vf/1
  Vref/1 -> Turbine  & Excitation Regulators Mac2/1(Pref)
  Turbine  & Excitation Regulators Mac2/1(Pm) -> Pm/1
  Pref1/1 -> Turbine  & Excitation Regulators Mac2/2(Vref)

== system GFo_29bus/North-West Network/Regulators3 ==
  m : Inport
  Bus Selector1 : BusSelector  OutputSignals="dq0 components.Stator voltage  vq (pu),dq0 components.Stator voltage  vd (pu),Mechanical.Rotor speed  wm  (pu),Output active power   Peo (pu)"
  Math Function1 : Math  Operator=hypot  SaturateOnIntegerOverflow=on
  Pref1 : Constant
  Turbine  & Excitation Regulators Mac2 : Subsystem
  Vref : Constant  Value=0.9
  Pm : Outport
  Vf : Outport  Port=2
  tag scope: Vm3=global, w3=global
  wires:
  Pref1/1 -> Turbine  & Excitation Regulators Mac2/2(Vref)
  Turbine  & Excitation Regulators Mac2/1(Pm) -> Pm/1
  Vref/1 -> Turbine  & Excitation Regulators Mac2/1(Pref)
  Turbine  & Excitation Regulators Mac2/2(Vf) -> Vf/1
  Bus Selector1/1 -> Math Function1/1  "<Stator voltage  vq (pu)>"
  Bus Selector1/2 -> Math Function1/2  "<Stator voltage  vd (pu)>"
  Math Function1/1 -> Turbine  & Excitation Regulators Mac2/3(Vm), [Vm3]
  Bus Selector1/3 -> Turbine  & Excitation Regulators Mac2/4(w), [w3]  "<Rotor speed  wm  (pu)>"
  Bus Selector1/4 -> Turbine  & Excitation Regulators Mac2/5(Pe)  "<Output active power   Peo (pu)>"
  m/1 -> Bus Selector1/1

== system GFo_29bus/North-West Network/Regulators4 ==
  m : Inport
  Bus Selector1 : BusSelector  OutputSignals="dq0 components.Stator voltage  vq (pu),dq0 components.Stator voltage  vd (pu),Mechanical.Rotor speed  wm  (pu),Output active power   Peo (pu)"
  Math Function1 : Math  Operator=hypot  SaturateOnIntegerOverflow=on
  Pref1 : Constant
  Turbine  & Excitation Regulators Mac2 : Subsystem
  Vref : Constant  Value=0.92593
  Pm : Outport
  Vf : Outport  Port=2
  tag scope: Vm4=global
  wires:
  m/1 -> Bus Selector1/1
  Bus Selector1/4 -> Turbine  & Excitation Regulators Mac2/5(Pe)  "<Output active power   Peo (pu)>"
  Bus Selector1/3 -> Turbine  & Excitation Regulators Mac2/4(w)  "<Rotor speed  wm  (pu)>"
  Math Function1/1 -> [Vm4], Turbine  & Excitation Regulators Mac2/3(Vm)
  Bus Selector1/2 -> Math Function1/2  "<Stator voltage  vd (pu)>"
  Bus Selector1/1 -> Math Function1/1  "<Stator voltage  vq (pu)>"
  Turbine  & Excitation Regulators Mac2/2(Vf) -> Vf/1
  Vref/1 -> Turbine  & Excitation Regulators Mac2/1(Pref)
  Turbine  & Excitation Regulators Mac2/1(Pm) -> Pm/1
  Pref1/1 -> Turbine  & Excitation Regulators Mac2/2(Vref)

== system GFo_29bus/North_East Network/Cs ARNS1  ==
  note: B
  Ca : powerlib/Elements/Series RLC Branch  LConnTagsString=__new0  RConnTagsString=__new0  BranchType=C  Resistance=1.0  Inductance=1.0  SetiL0=off  InitialCurrent=0  Capacitance=Cs  Setx0=off  InitialVoltage=0  Measurements=None
  Cb : powerlib/Elements/Series RLC Branch  LConnTagsString=__new0  RConnTagsString=__new0  BranchType=C  Resistance=1.0  Inductance=1.0  SetiL0=off  InitialCurrent=0  Capacitance=Cs  Setx0=off  InitialVoltage=0  Measurements=None
  Cc : powerlib/Elements/Series RLC Branch  LConnTagsString=__new0  RConnTagsString=__new0  BranchType=C  Resistance=1.0  Inductance=1.0  SetiL0=off  InitialCurrent=0  Capacitance=Cs  Setx0=off  InitialVoltage=0  Measurements=None
  A : PMIOPort  Port=1  Side=Left
  B : PMIOPort  Port=2  Side=Left
  C : PMIOPort  Port=3  Side=Left
  "A " : PMIOPort  Port=4  Side=Right
  "B " : PMIOPort  Port=5  Side=Right
  "C " : PMIOPort  Port=6  Side=Right
  connections:
  Cc/RConn1 -- "C "/RConn1
  C/RConn1 -- Cc/LConn1
  Cb/RConn1 -- "B "/RConn1
  B/RConn1 -- Cb/LConn1
  Ca/RConn1 -- "A "/RConn1
  A/RConn1 -- Ca/LConn1

== system GFo_29bus/North_East Network/Cs ARNS2 ==
  note: B
  Ca : powerlib/Elements/Series RLC Branch  LConnTagsString=__new0  RConnTagsString=__new0  BranchType=C  Resistance=1.0  Inductance=1.0  SetiL0=off  InitialCurrent=0  Capacitance=Cs  Setx0=off  InitialVoltage=0  Measurements=None
  Cb : powerlib/Elements/Series RLC Branch  LConnTagsString=__new0  RConnTagsString=__new0  BranchType=C  Resistance=1.0  Inductance=1.0  SetiL0=off  InitialCurrent=0  Capacitance=Cs  Setx0=off  InitialVoltage=0  Measurements=None
  Cc : powerlib/Elements/Series RLC Branch  LConnTagsString=__new0  RConnTagsString=__new0  BranchType=C  Resistance=1.0  Inductance=1.0  SetiL0=off  InitialCurrent=0  Capacitance=Cs  Setx0=off  InitialVoltage=0  Measurements=None
  A : PMIOPort  Port=1  Side=Left
  B : PMIOPort  Port=2  Side=Left
  C : PMIOPort  Port=3  Side=Left
  "A " : PMIOPort  Port=4  Side=Right
  "B " : PMIOPort  Port=5  Side=Right
  "C " : PMIOPort  Port=6  Side=Right
  connections:
  A/RConn1 -- Ca/LConn1
  Ca/RConn1 -- "A "/RConn1
  B/RConn1 -- Cb/LConn1
  Cb/RConn1 -- "B "/RConn1
  C/RConn1 -- Cc/LConn1
  Cc/RConn1 -- "C "/RConn1

== system GFo_29bus/North_East Network/Cs BER ==
  note: B
  Ca : powerlib/Elements/Series RLC Branch  LConnTagsString=__new0  RConnTagsString=__new0  BranchType=C  Resistance=1.0  Inductance=1.0  SetiL0=off  InitialCurrent=0  Capacitance=Cs  Setx0=off  InitialVoltage=0  Measurements=None
  Cb : powerlib/Elements/Series RLC Branch  LConnTagsString=__new0  RConnTagsString=__new0  BranchType=C  Resistance=1.0  Inductance=1.0  SetiL0=off  InitialCurrent=0  Capacitance=Cs  Setx0=off  InitialVoltage=0  Measurements=None
  Cc : powerlib/Elements/Series RLC Branch  LConnTagsString=__new0  RConnTagsString=__new0  BranchType=C  Resistance=1.0  Inductance=1.0  SetiL0=off  InitialCurrent=0  Capacitance=Cs  Setx0=off  InitialVoltage=0  Measurements=None
  A : PMIOPort  Port=1  Side=Left
  B : PMIOPort  Port=2  Side=Left
  C : PMIOPort  Port=3  Side=Left
  "A " : PMIOPort  Port=4  Side=Right
  "B " : PMIOPort  Port=5  Side=Right
  "C " : PMIOPort  Port=6  Side=Right
  connections:
  Cc/RConn1 -- "C "/RConn1
  C/RConn1 -- Cc/LConn1
  Cb/RConn1 -- "B "/RConn1
  B/RConn1 -- Cb/LConn1
  Ca/RConn1 -- "A "/RConn1
  A/RConn1 -- Ca/LConn1

== system GFo_29bus/North_East Network/Cs MTG+ARNN  ==
  note: B
  Ca : powerlib/Elements/Series RLC Branch  LConnTagsString=__new0  RConnTagsString=__new0  BranchType=C  Resistance=1.0  Inductance=1.0  SetiL0=off  InitialCurrent=0  Capacitance=Cs  Setx0=off  InitialVoltage=0  Measurements=None
  Cb : powerlib/Elements/Series RLC Branch  LConnTagsString=__new0  RConnTagsString=__new0  BranchType=C  Resistance=1.0  Inductance=1.0  SetiL0=off  InitialCurrent=0  Capacitance=Cs  Setx0=off  InitialVoltage=0  Measurements=None
  Cc : powerlib/Elements/Series RLC Branch  LConnTagsString=__new0  RConnTagsString=__new0  BranchType=C  Resistance=1.0  Inductance=1.0  SetiL0=off  InitialCurrent=0  Capacitance=Cs  Setx0=off  InitialVoltage=0  Measurements=None
  A : PMIOPort  Port=1  Side=Left
  B : PMIOPort  Port=2  Side=Left
  C : PMIOPort  Port=3  Side=Left
  "A " : PMIOPort  Port=4  Side=Right
  "B " : PMIOPort  Port=5  Side=Right
  "C " : PMIOPort  Port=6  Side=Right
  connections:
  A/RConn1 -- Ca/LConn1
  Ca/RConn1 -- "A "/RConn1
  B/RConn1 -- Cb/LConn1
  Cb/RConn1 -- "B "/RConn1
  C/RConn1 -- Cc/LConn1
  Cc/RConn1 -- "C "/RConn1

== system GFo_29bus/North_East Network/Cs PER  ==
  note: B
  Ca : powerlib/Elements/Series RLC Branch  LConnTagsString=__new0  RConnTagsString=__new0  BranchType=C  Resistance=1.0  Inductance=1.0  SetiL0=off  InitialCurrent=0  Capacitance=Cs  Setx0=off  InitialVoltage=0  Measurements=None
  Cb : powerlib/Elements/Series RLC Branch  LConnTagsString=__new0  RConnTagsString=__new0  BranchType=C  Resistance=1.0  Inductance=1.0  SetiL0=off  InitialCurrent=0  Capacitance=Cs  Setx0=off  InitialVoltage=0  Measurements=None
  Cc : powerlib/Elements/Series RLC Branch  LConnTagsString=__new0  RConnTagsString=__new0  BranchType=C  Resistance=1.0  Inductance=1.0  SetiL0=off  InitialCurrent=0  Capacitance=Cs  Setx0=off  InitialVoltage=0  Measurements=None
  A : PMIOPort  Port=1  Side=Left
  B : PMIOPort  Port=2  Side=Left
  C : PMIOPort  Port=3  Side=Left
  "A " : PMIOPort  Port=4  Side=Right
  "B " : PMIOPort  Port=5  Side=Right
  "C " : PMIOPort  Port=6  Side=Right
  connections:
  A/RConn1 -- Ca/LConn1
  Ca/RConn1 -- "A "/RConn1
  B/RConn1 -- Cb/LConn1
  Cb/RConn1 -- "B "/RConn1
  C/RConn1 -- Cc/LConn1
  Cc/RConn1 -- "C "/RConn1

== system GFo_29bus/North_East Network/Regulateurs6 ==
  m : Inport
  Bus Selector1 : BusSelector  OutputSignals="dq0 components.Stator voltage  vq (pu),dq0 components.Stator voltage  vd (pu),Mechanical.Rotor speed  wm  (pu),Output active power   Peo (pu)"
  Math Function1 : Math  Operator=hypot  SaturateOnIntegerOverflow=on
  Pref1 : Constant
  Turbine  & Excitation Regulators Mac2 : Subsystem
  Vref : Constant  Value=0.89286
  Pm : Outport
  Vf : Outport  Port=2
  tag scope: Vm6=global, w6=global
  wires:
  Pref1/1 -> Turbine  & Excitation Regulators Mac2/2(Vref)
  Turbine  & Excitation Regulators Mac2/1(Pm) -> Pm/1
  Vref/1 -> Turbine  & Excitation Regulators Mac2/1(Pref)
  Turbine  & Excitation Regulators Mac2/2(Vf) -> Vf/1
  Bus Selector1/1 -> Math Function1/1  "<Stator voltage  vq (pu)>"
  Bus Selector1/2 -> Math Function1/2  "<Stator voltage  vd (pu)>"
  Math Function1/1 -> Turbine  & Excitation Regulators Mac2/3(Vm), [Vm6]
  Bus Selector1/3 -> Turbine  & Excitation Regulators Mac2/4(w), [w6]  "<Rotor speed  wm  (pu)>"
  Bus Selector1/4 -> Turbine  & Excitation Regulators Mac2/5(Pe)  "<Output active power   Peo (pu)>"
  m/1 -> Bus Selector1/1

== system GFo_29bus/North_East Network/Regulateurs7 ==
  m : Inport
  Bus Selector1 : BusSelector  OutputSignals="dq0 components.Stator voltage  vq (pu),dq0 components.Stator voltage  vd (pu),Mechanical.Rotor speed  wm  (pu),Output active power   Peo (pu)"
  Math Function1 : Math  Operator=hypot  SaturateOnIntegerOverflow=on
  Pref1 : Constant
  Turbine  & Excitation Regulators Mac2 : Subsystem
  Vref : Constant  Value=0.9
  Pm : Outport
  Vf : Outport  Port=2
  tag scope: Vm7=global, w7=global
  wires:
  m/1 -> Bus Selector1/1
  Bus Selector1/4 -> Turbine  & Excitation Regulators Mac2/5(Pe)  "<Output active power   Peo (pu)>"
  Bus Selector1/3 -> Turbine  & Excitation Regulators Mac2/4(w), [w7]  "<Rotor speed  wm  (pu)>"
  Math Function1/1 -> [Vm7], Turbine  & Excitation Regulators Mac2/3(Vm)
  Bus Selector1/2 -> Math Function1/2  "<Stator voltage  vd (pu)>"
  Bus Selector1/1 -> Math Function1/1  "<Stator voltage  vq (pu)>"
  Turbine  & Excitation Regulators Mac2/2(Vf) -> Vf/1
  Vref/1 -> Turbine  & Excitation Regulators Mac2/1(Pref)
  Turbine  & Excitation Regulators Mac2/1(Pm) -> Pm/1
  Pref1/1 -> Turbine  & Excitation Regulators Mac2/2(Vref)

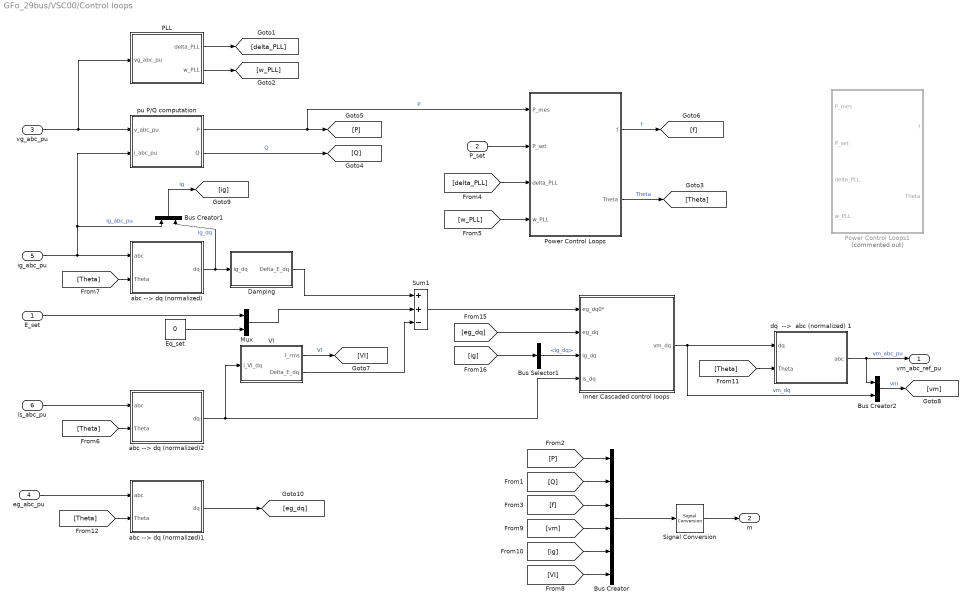
== system GFo_29bus/VSC00/Control loops ==
  E_set : Inport
  P_set : Inport  Port=2
  vg_abc_pu : Inport  Port=3
  eg_abc_pu : Inport  Port=4
  ig_abc_pu : Inport  Port=5
  is_abc_pu : Inport  Port=6
  " pu P/Q computation" : Subsystem  DialogController=POWERSYS.PowerSysDialog
  Bus Creator : BusCreator  Inputs=6
  Bus Creator1 : BusCreator  Inputs=2
  Bus Creator2 : BusCreator  Inputs=2
  Bus Selector1 : BusSelector  OutputSignals=ig_dq
  Damping : Subsystem
  Eq_set : Constant  Value=0
  Inner Cascaded control loops : Subsystem
  Mux : Mux  Inputs=2
  PLL : Subsystem
  Power Control Loops : Subsystem
  Power Control Loops1 : Subsystem  Commented=on
  Signal Conversion : SignalConversion  OverrideOpt=off
  Sum1 : Sum  Inputs=++-
  VI : Subsystem
  abc --> dq (normalized) : Subsystem
  abc --> dq (normalized)1 : Subsystem
  abc --> dq (normalized)2 : Subsystem
  dq  -->  abc (normalized) 1 : Subsystem
  vm_abc_ref_pu : Outport
  m : Outport  Port=2
  wires:
  Signal Conversion/1 -> m/1
  [P] -> Bus Creator/1
  [Q] -> Bus Creator/2
  [f] -> Bus Creator/3
  E_set/1 -> Mux/1
  " pu P/Q computation"/2(Q) -> [Q]  "Q"
  [delta_PLL] -> Power Control Loops/3(delta_PLL)
  P_set/1 -> Power Control Loops/2(P_set)
  [w_PLL] -> Power Control Loops/4(w_PLL)
  Power Control Loops/1(f) -> [f]  "f"
  PLL/1(delta_PLL) -> [delta_PLL]
  PLL/2(w_PLL) -> [w_PLL]
  " pu P/Q computation"/1(P) -> Power Control Loops/1(P_mes), [P]  "P"
  ig_abc_pu/1 -> Bus Creator1/1, " pu P/Q computation"/2(i_abc_pu), abc --> dq (normalized)/1(abc)  "ig_abc_pu"
  abc --> dq (normalized)/1(dq) -> Damping/1(ig_dq), Bus Creator1/2  "ig_dq"
  Power Control Loops/2(Theta) -> [Theta]  "Theta"
  [Theta] -> abc --> dq (normalized)/2(Theta)
  VI/2(Delta_E_dq) -> Sum1/3
  Damping/1("Delta_E_dq ") -> Sum1/1
  VI/1(I_rms) -> [VI]  "VI"
  Mux/1 -> Sum1/2
  Eq_set/1 -> Mux/2
  [vm] -> Bus Creator/4
  [VI] -> Bus Creator/6
  Bus Creator/1 -> Signal Conversion/1
  Bus Creator1/1 -> [ig]  "ig"
  [ig] -> Bus Creator/5
  [Theta] -> abc --> dq (normalized)2/2(Theta)
  vg_abc_pu/1 -> PLL/1(vg_abc_pu), " pu P/Q computation"/1(v_abc_pu)
  abc --> dq (normalized)2/1(dq) -> Inner Cascaded control loops/4(is_dq), VI/1(i_VI_dq)
  [Theta] -> abc --> dq (normalized)1/2(Theta)
  abc --> dq (normalized)1/1(dq) -> [eg_dq]
  is_abc_pu/1 -> abc --> dq (normalized)2/1(abc)
  eg_abc_pu/1 -> abc --> dq (normalized)1/1(abc)
  [eg_dq] -> Inner Cascaded control loops/2(eg_dq)
  Inner Cascaded control loops/1(vm_dq) -> dq  -->  abc (normalized) 1/1(dq), Bus Creator2/2  "vm_dq"
  dq  -->  abc (normalized) 1/1(abc) -> Bus Creator2/1, vm_abc_ref_pu/1  "vm_abc_pu"
  [Theta] -> dq  -->  abc (normalized) 1/2(Theta)
  Bus Creator2/1 -> [vm]  "vm"
  Bus Selector1/1 -> Inner Cascaded control loops/3(ig_dq)  "<ig_dq>"
  [ig] -> Bus Selector1/1
  Sum1/1 -> Inner Cascaded control loops/1(eg_dq0*)

== system GFo_29bus/VSC00/Mean_model ==
  Uref : Inport
  NOT1 : Logic  Operator=NOT  IconShape=distinctive  AllPortsSameDT=off  OutDataTypeStr=boolean
  Scope : Scope
  Step1 : Step  Time=Time_Step  SampleTime=Time_Step
  Three-Phase Breaker1 : powerlib/Elements/Three-Phase Breaker  InitialState=closed  SwitchA=on  SwitchB=on  SwitchC=on  SwitchTimes="[4/60  10/60]"  External=on  BreakerResistance=0.001  SnubberResistance=1e6  SnubberCapacitance=inf  Measurements=None
  Three-Phase Breaker2 : powerlib/Elements/Three-Phase Breaker  InitialState=open  SwitchA=on  SwitchB=on  SwitchC=on  SwitchTimes="[4/60  10/60]"  External=on  BreakerResistance=0.001  SnubberResistance=1e6  SnubberCapacitance=inf  Measurements=None
  Three-Phase Source : powerlib/Electrical Sources/Three-Phase Source  InternalConnection=Yg  VoltagePhases=off  Voltage=Vvsc0*Un1  PhaseAngle=Theta_vsc0  Voltage_phases=[25e3 25e3 25e3]/sqrt(3)  PhaseAngles_phases=[0 -120 +120]  Frequency=fb  NonIdealSource=off  SpecifyImpedance=off  Resistance=0  Inductance=0  ShortCircuitLevel=100e6  BaseVoltage=VSC01_Un1  XRratio=7  BusType=swing  Pref=0.3  Qref=0  Prefabc=[10e3, 10e3, 10e3]  Qrefabc=[0, 0, 0]  Qmin=-Inf  Qmax=Inf
  Universal Bridge : powerlib/Power Electronics/Universal Bridge  Arms=3  SnubberResistance=1e5  SnubberCapacitance=inf  Device=Average-model based VSC  Ron=1e-3  Lon=0  ForwardVoltages="[  0  0  ]"  ForwardVoltage=0  GTOparameters=[ 10e-6 , 20e-6 ]  IGBTparameters=[ 1e-6 , 2e-6 ]  Measurements=None  Measurements_2=None  converterType=Rectifier
  Vdc : powerlib/Measurements/Voltage Measurement  PhasorSimulation=off  OutputType=Complex  PSBequivalent=0
  mp3 : Gain  Gain=2/VSC01_Udcb
  PhA : PMIOPort  Port=1  Side=Right
  PhB : PMIOPort  Port=2  Side=Right
  PhC : PMIOPort  Port=3  Side=Right
  Vdc+ : PMIOPort  Port=4  Side=Left
  Vdc- : PMIOPort  Port=5  Side=Left
  wires:
  Vdc/1 -> Scope/1
  Uref/1 -> mp3/1
  mp3/1 -> Universal Bridge/1
  Step1/1 -> Three-Phase Breaker2/1, NOT1/1
  NOT1/1 -> Three-Phase Breaker1/1
  connections:
  Vdc-/RConn1 -- Universal Bridge/RConn2 -- Vdc/LConn2
  Vdc+/RConn1 -- Universal Bridge/RConn1 -- Vdc/LConn1
  Three-Phase Source/RConn3 -- Three-Phase Breaker1/RConn3
  Three-Phase Source/RConn2 -- Three-Phase Breaker1/RConn2
  Three-Phase Source/RConn1 -- Three-Phase Breaker1/RConn1
  Three-Phase Breaker2/RConn3 -- Universal Bridge/LConn3
  Three-Phase Breaker2/RConn2 -- Universal Bridge/LConn2
  Three-Phase Breaker2/RConn1 -- Universal Bridge/LConn1
  PhC/RConn1 -- Three-Phase Breaker1/LConn3 -- Three-Phase Breaker2/LConn3
  PhB/RConn1 -- Three-Phase Breaker1/LConn2 -- Three-Phase Breaker2/LConn2
  PhA/RConn1 -- Three-Phase Breaker1/LConn1 -- Three-Phase Breaker2/LConn1

== system GFo_29bus/VSC00/Output_Filter ==
  Filter capacitance : powerlib/Elements/Three-Phase Series RLC Branch  LConnTagsString=A|B|C  RConnTagsString=A|B|C  BranchType=C  Resistance=0  Inductance=C_line(1)  Capacitance=Cf_pu*Cb  Measurements=None
  Filter inductance : powerlib/Elements/Three-Phase Series RLC Branch  LConnTagsString=A|B|C  RConnTagsString=A|B|C  BranchType=RL  Resistance=Rf_pu*Zb  Inductance=Lf_pu*Lb  Capacitance=1e-6  Measurements=None
  Ground : powerlib/Elements/Ground  LConnTagsString=a
  A : PMIOPort  Port=1  Side=Left
  a : PMIOPort  Port=2  Side=Right
  B : PMIOPort  Port=3  Side=Left
  b : PMIOPort  Port=4  Side=Right
  C : PMIOPort  Port=5  Side=Left
  c : PMIOPort  Port=6  Side=Right
  connections:
  Filter inductance/RConn1 -- Filter capacitance/LConn1 -- a/RConn1
  Filter inductance/RConn3 -- Filter capacitance/LConn3 -- c/RConn1
  Filter inductance/LConn2 -- B/RConn1
  Filter inductance/LConn3 -- C/RConn1
  Filter inductance/LConn1 -- A/RConn1
  Filter inductance/RConn2 -- Filter capacitance/LConn2 -- b/RConn1
  Filter capacitance/RConn2 -- Filter capacitance/RConn3 -- Filter capacitance/RConn1 -- Ground/LConn1

== system GFo_29bus/North-West Network/Regulators1/Turbine  & Excitation Regulators Mac2 ==
  Pref : Inport
  Vref : Inport  Port=2
  Vm : Inport  Port=3
  w : Inport  Port=4
  Pe : Inport  Port=5
  Add : Sum  Inputs=+-
  Complex to Real-Imag : ComplexToRealImag
  Excitation System : sps_avr/Excitation System  tr=20e-3  reg=[ 300, 0.001 ]  exc=[ 1, 0 ]  tgr=[ 0, 0 ]  damp=[ 0.001, 0.1 ]  sat=[ 0, 0 ]  lim=[ -11.5, 11.5, 0 ]  v0=[1 1.3813]
  Hydraulic Turbine and Governor : powerlib/Machines/Hydraulic Turbine and Governor  sm="[ 10/3  0.07 ]"  gate="[  0.01  0.97518  -0.1  0.1 ]"  reg="[  0.05 1.163  0.105  0  0.01  ]"  hyd="[  0  2.67  ]"  dref=0  po=0.91213
  Stabilisateur : Subsystem
  Terminator : Terminator
  wref : Constant
  wref1 : Constant
  Pm : Outport
  Vf : Outport  Port=2
  wires:
  Hydraulic Turbine and Governor/2 -> Terminator/1
  Hydraulic Turbine and Governor/1 -> Pm/1, Stabilisateur/1(Pm)
  Excitation System/1 -> Vf/1
  Pe/1 -> Hydraulic Turbine and Governor/4, Stabilisateur/2(Pe)
  Pref/1 -> Hydraulic Turbine and Governor/2
  Vref/1 -> Excitation System/1
  wref/1 -> Hydraulic Turbine and Governor/1
  w/1 -> Hydraulic Turbine and Governor/3, Add/1
  Vm/1 -> Complex to Real-Imag/1
  Complex to Real-Imag/2 -> Excitation System/3
  Complex to Real-Imag/1 -> Excitation System/2
  wref1/1 -> Add/2
  Add/1 -> Hydraulic Turbine and Governor/5, Stabilisateur/3(dw)
  Stabilisateur/1(Stab) -> Excitation System/4

== system GFo_29bus/North-West Network/Regulators2/Turbine  & Excitation Regulators Mac2 ==
  Pref : Inport
  Vref : Inport  Port=2
  Vm : Inport  Port=3
  w : Inport  Port=4
  Pe : Inport  Port=5
  Add : Sum  Inputs=+-
  Complex to Real-Imag : ComplexToRealImag
  Excitation System : sps_avr/Excitation System  tr=20e-3  reg=[ 300, 0.001 ]  exc=[ 1, 0 ]  tgr=[ 0, 0 ]  damp=[ 0.001, 0.1 ]  sat=[ 0, 0 ]  lim=[ -11.5, 11.5, 0 ]  v0=[1 1.3735]
  Hydraulic Turbine and Governor : powerlib/Machines/Hydraulic Turbine and Governor  sm="[ 10/3  0.07 ]"  gate="[  0.01  0.97518  -0.1  0.1 ]"  reg="[  0.05 1.163  0.105  0  0.01  ]"  hyd="[  0  2.67  ]"  dref=0  po=0.8201
  Stabilisateur : Subsystem
  Terminator : Terminator
  wref : Constant
  wref1 : Constant
  Pm : Outport
  Vf : Outport  Port=2
  wires:
  Stabilisateur/1(Stab) -> Excitation System/4
  Add/1 -> Stabilisateur/3(dw), Hydraulic Turbine and Governor/5
  wref1/1 -> Add/2
  Complex to Real-Imag/1 -> Excitation System/2
  Complex to Real-Imag/2 -> Excitation System/3
  Vm/1 -> Complex to Real-Imag/1
  w/1 -> Add/1, Hydraulic Turbine and Governor/3
  wref/1 -> Hydraulic Turbine and Governor/1
  Vref/1 -> Excitation System/1
  Pref/1 -> Hydraulic Turbine and Governor/2
  Pe/1 -> Stabilisateur/2(Pe), Hydraulic Turbine and Governor/4
  Excitation System/1 -> Vf/1
  Hydraulic Turbine and Governor/1 -> Stabilisateur/1(Pm), Pm/1
  Hydraulic Turbine and Governor/2 -> Terminator/1

== system GFo_29bus/North-West Network/Regulators3/Turbine  & Excitation Regulators Mac2 ==
  Pref : Inport
  Vref : Inport  Port=2
  Vm : Inport  Port=3
  w : Inport  Port=4
  Pe : Inport  Port=5
  Add : Sum  Inputs=+-
  Complex to Real-Imag : ComplexToRealImag
  Excitation System : sps_avr/Excitation System  tr=20e-3  reg=[ 300, 0.001 ]  exc=[ 1, 0 ]  tgr=[ 0, 0 ]  damp=[ 0.001, 0.1 ]  sat=[ 0, 0 ]  lim=[ -11.5, 11.5, 0 ]  v0=[1 1.44]
  Hydraulic Turbine and Governor : powerlib/Machines/Hydraulic Turbine and Governor  sm="[ 10/3  0.07 ]"  gate="[  0.01  0.97518  -0.1  0.1 ]"  reg="[  0.05 1.163  0.105  0  0.01  ]"  hyd="[  0  2.67  ]"  dref=0  po=0.90232
  Stabilisateur : Subsystem
  Terminator : Terminator
  wref : Constant
  wref1 : Constant
  Pm : Outport
  Vf : Outport  Port=2
  wires:
  Hydraulic Turbine and Governor/2 -> Terminator/1
  Hydraulic Turbine and Governor/1 -> Pm/1, Stabilisateur/1(Pm)
  Excitation System/1 -> Vf/1
  Pe/1 -> Hydraulic Turbine and Governor/4, Stabilisateur/2(Pe)
  Pref/1 -> Hydraulic Turbine and Governor/2
  Vref/1 -> Excitation System/1
  wref/1 -> Hydraulic Turbine and Governor/1
  w/1 -> Hydraulic Turbine and Governor/3, Add/1
  Vm/1 -> Complex to Real-Imag/1
  Complex to Real-Imag/2 -> Excitation System/3
  Complex to Real-Imag/1 -> Excitation System/2
  wref1/1 -> Add/2
  Add/1 -> Hydraulic Turbine and Governor/5, Stabilisateur/3(dw)
  Stabilisateur/1(Stab) -> Excitation System/4

== system GFo_29bus/North-West Network/Regulators4/Turbine  & Excitation Regulators Mac2 ==
  Pref : Inport
  Vref : Inport  Port=2
  Vm : Inport  Port=3
  w : Inport  Port=4
  Pe : Inport  Port=5
  Add : Sum  Inputs=+-
  Complex to Real-Imag : ComplexToRealImag
  Excitation System : sps_avr/Excitation System  tr=20e-3  reg=[ 300, 0.001 ]  exc=[ 1, 0 ]  tgr=[ 0, 0 ]  damp=[ 0.001, 0.1 ]  sat=[ 0, 0 ]  lim=[ -11.5, 11.5, 0 ]  v0=[1 1.3734]
  Hydraulic Turbine and Governor : powerlib/Machines/Hydraulic Turbine and Governor  sm="[ 10/3  0.07 ]"  gate="[  0.01  0.97518  -0.1  0.1 ]"  reg="[  0.05 1.163  0.105  0  0.01  ]"  hyd="[  0  2.67  ]"  dref=0  po=0.92838
  Stabilisateur : Subsystem
  Terminator : Terminator
  wref : Constant
  wref1 : Constant
  Pm : Outport
  Vf : Outport  Port=2
  wires:
  Stabilisateur/1(Stab) -> Excitation System/4
  Add/1 -> Stabilisateur/3(dw), Hydraulic Turbine and Governor/5
  wref1/1 -> Add/2
  Complex to Real-Imag/1 -> Excitation System/2
  Complex to Real-Imag/2 -> Excitation System/3
  Vm/1 -> Complex to Real-Imag/1
  w/1 -> Add/1, Hydraulic Turbine and Governor/3
  wref/1 -> Hydraulic Turbine and Governor/1
  Vref/1 -> Excitation System/1
  Pref/1 -> Hydraulic Turbine and Governor/2
  Pe/1 -> Stabilisateur/2(Pe), Hydraulic Turbine and Governor/4
  Excitation System/1 -> Vf/1
  Hydraulic Turbine and Governor/1 -> Stabilisateur/1(Pm), Pm/1
  Hydraulic Turbine and Governor/2 -> Terminator/1
